simulink model "p1c1"  (R2023b)
settings: Solver=VariableStepAuto  StartTime=0.0  StopTime=30  RelTol=1e-3
settings Model: Creator=tanvi  LastModifiedBy=m96sz

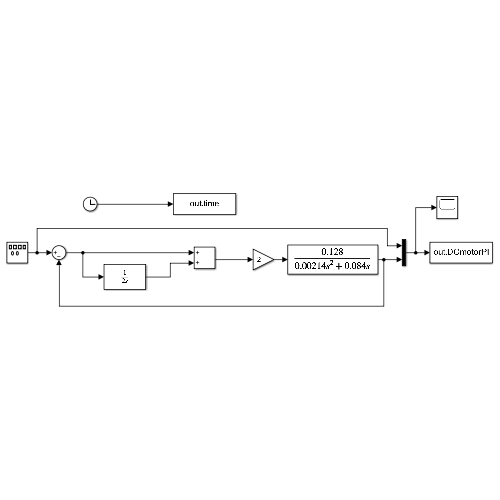
[thumbnail: Simulink's stored preview of the top-level diagram]
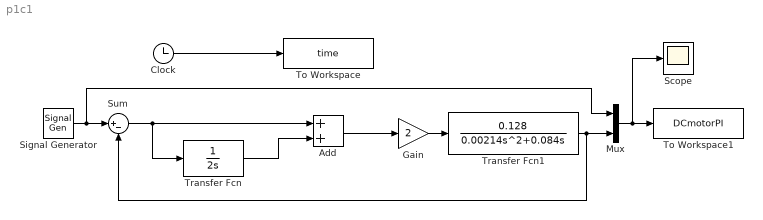
== system p1c1 ==
  Add : Sum
  Clock : Clock
  Gain : Gain  Gain=2
  Mux : Mux  Inputs=2
  Scope : Scope
  Signal Generator : SignalGenerator  WaveForm=sawtooth  Frequency=0.1
  Sum : Sum  Inputs=|+-
  To Workspace : ToWorkspace  VariableName=time  SampleTime=-1
  To Workspace1 : ToWorkspace  VariableName=DCmotorPI  SampleTime=-1
  Transfer Fcn : TransferFcn  Denominator=[2 0]
  Transfer Fcn1 : TransferFcn  Numerator=[0.128]  Denominator=[0.00214 0.084 0]
  wires:
  Clock/1 -> To Workspace/1
  Gain/1 -> Transfer Fcn1/1
  Mux/1 -> Scope/1, To Workspace1/1
  Add/1 -> Gain/1
  Transfer Fcn/1 -> Add/2
  Transfer Fcn1/1 -> Sum/2, Mux/2
  Sum/1 -> Transfer Fcn/1, Add/1
  Signal Generator/1 -> Mux/1, Sum/1
